simulink model "bu01_2018b"  (R2018b)
settings: Solver=VariableStepAuto  StartTime=0.0  StopTime=10.0  RelTol=1e-3
model workspace (MAT data in the model file):
  Ixx = 0.8
  Iyy = 2.075
  Izz = 1.25
  Mass = 11.5
libraries: aerolibutil x6, sharedtransform x4, simulink x3, sharedutil x3, shared6dof x1
(part 2 of 2)

== system bu01_2018b/bu01_model/推力方程/动力模型/螺旋桨模型1 ==
  u1 : Inport
  Add : Sum  Inputs=4
  Constant : Constant  Value=0
  Constant1 : Constant  Value=0.1591
  Constant2 : Constant  Value=0.1591
  Constant3 : Constant  Value=0.3295
  Constant4 : Constant  Value=0.3295
  Constant5 : Constant  Value=0.7273
  Constant6 : Constant  Value=0.7273
  Constant7 : Constant  Value=1.0
  Gain : Gain  Gain=0.2196
  Gain1 : Gain  Gain=514.4904
  Gain2 : Gain  Gain=2.6589e+03
  Gain3 : Gain  Gain=317.0137
  MATLAB Function : MATLAB Function  TreatAsAtomicUnit=on
  MATLAB Function1 : MATLAB Function  TreatAsAtomicUnit=on
  MATLAB Function2 : MATLAB Function  TreatAsAtomicUnit=on
  MATLAB Function3 : MATLAB Function  TreatAsAtomicUnit=on
  Out1 : Outport
  wires:
  Add/1 -> Out1/1
  u1/1 -> MATLAB Function1/1(u), MATLAB Function/1(u), MATLAB Function2/1(u), MATLAB Function3/1(u)
  Gain3/1 -> Add/4
  Gain2/1 -> Add/3
  Gain1/1 -> Add/2
  Gain/1 -> Add/1
  Constant7/1 -> MATLAB Function3/3(b)
  Constant6/1 -> MATLAB Function3/2(a)
  Constant5/1 -> MATLAB Function2/3(b)
  Constant4/1 -> MATLAB Function2/2(a)
  Constant3/1 -> MATLAB Function1/3(b)
  Constant2/1 -> MATLAB Function1/2(a)
  Constant1/1 -> MATLAB Function/3(b)
  Constant/1 -> MATLAB Function/2(a)
  MATLAB Function3/1(y) -> Gain3/1
  MATLAB Function2/1(y) -> Gain2/1
  MATLAB Function1/1(y) -> Gain1/1
  MATLAB Function/1(y) -> Gain/1

== system bu01_2018b/bu01_model/推力方程/动力模型/螺旋桨模型2 ==
  u1 : Inport
  Add : Sum  Inputs=4
  Constant : Constant  Value=0
  Constant1 : Constant  Value=0.1591
  Constant2 : Constant  Value=0.1591
  Constant3 : Constant  Value=0.3295
  Constant4 : Constant  Value=0.3295
  Constant5 : Constant  Value=0.7273
  Constant6 : Constant  Value=0.7273
  Constant7 : Constant  Value=1.0
  Gain : Gain  Gain=0.2196
  Gain1 : Gain  Gain=514.4904
  Gain2 : Gain  Gain=2.6589e+03
  Gain3 : Gain  Gain=317.0137
  MATLAB Function : MATLAB Function  TreatAsAtomicUnit=on
  MATLAB Function1 : MATLAB Function  TreatAsAtomicUnit=on
  MATLAB Function2 : MATLAB Function  TreatAsAtomicUnit=on
  MATLAB Function3 : MATLAB Function  TreatAsAtomicUnit=on
  Out1 : Outport
  wires:
  MATLAB Function/1(y) -> Gain/1
  MATLAB Function1/1(y) -> Gain1/1
  MATLAB Function2/1(y) -> Gain2/1
  MATLAB Function3/1(y) -> Gain3/1
  Constant/1 -> MATLAB Function/2(a)
  Constant1/1 -> MATLAB Function/3(b)
  Constant2/1 -> MATLAB Function1/2(a)
  Constant3/1 -> MATLAB Function1/3(b)
  Constant4/1 -> MATLAB Function2/2(a)
  Constant5/1 -> MATLAB Function2/3(b)
  Constant6/1 -> MATLAB Function3/2(a)
  Constant7/1 -> MATLAB Function3/3(b)
  Gain/1 -> Add/1
  Gain1/1 -> Add/2
  Gain2/1 -> Add/3
  Gain3/1 -> Add/4
  u1/1 -> MATLAB Function3/1(u), MATLAB Function2/1(u), MATLAB Function/1(u), MATLAB Function1/1(u)
  Add/1 -> Out1/1

== system bu01_2018b/bu01_model/推力方程/动力模型/螺旋桨模型3 ==
  u1 : Inport
  Add : Sum  Inputs=4
  Constant : Constant  Value=0
  Constant1 : Constant  Value=0.1591
  Constant2 : Constant  Value=0.1591
  Constant3 : Constant  Value=0.3295
  Constant4 : Constant  Value=0.3295
  Constant5 : Constant  Value=0.7273
  Constant6 : Constant  Value=0.7273
  Constant7 : Constant  Value=1.0
  Gain : Gain  Gain=0.2196
  Gain1 : Gain  Gain=514.4904
  Gain2 : Gain  Gain=2.6589e+03
  Gain3 : Gain  Gain=317.0137
  MATLAB Function : MATLAB Function  TreatAsAtomicUnit=on
  MATLAB Function1 : MATLAB Function  TreatAsAtomicUnit=on
  MATLAB Function2 : MATLAB Function  TreatAsAtomicUnit=on
  MATLAB Function3 : MATLAB Function  TreatAsAtomicUnit=on
  Out1 : Outport
  wires:
  Add/1 -> Out1/1
  u1/1 -> MATLAB Function1/1(u), MATLAB Function/1(u), MATLAB Function2/1(u), MATLAB Function3/1(u)
  Gain3/1 -> Add/4
  Gain2/1 -> Add/3
  Gain1/1 -> Add/2
  Gain/1 -> Add/1
  Constant7/1 -> MATLAB Function3/3(b)
  Constant6/1 -> MATLAB Function3/2(a)
  Constant5/1 -> MATLAB Function2/3(b)
  Constant4/1 -> MATLAB Function2/2(a)
  Constant3/1 -> MATLAB Function1/3(b)
  Constant2/1 -> MATLAB Function1/2(a)
  Constant1/1 -> MATLAB Function/3(b)
  Constant/1 -> MATLAB Function/2(a)
  MATLAB Function3/1(y) -> Gain3/1
  MATLAB Function2/1(y) -> Gain2/1
  MATLAB Function1/1(y) -> Gain1/1
  MATLAB Function/1(y) -> Gain/1

== system bu01_2018b/bu01_model/推力方程/动力模型/螺旋桨模型4 ==
  u1 : Inport
  Add : Sum  Inputs=4
  Constant : Constant  Value=0
  Constant1 : Constant  Value=0.1591
  Constant2 : Constant  Value=0.1591
  Constant3 : Constant  Value=0.3295
  Constant4 : Constant  Value=0.3295
  Constant5 : Constant  Value=0.7273
  Constant6 : Constant  Value=0.7273
  Constant7 : Constant  Value=1.0
  Gain : Gain  Gain=0.2196
  Gain1 : Gain  Gain=514.4904
  Gain2 : Gain  Gain=2.6589e+03
  Gain3 : Gain  Gain=317.0137
  MATLAB Function : MATLAB Function  TreatAsAtomicUnit=on
  MATLAB Function1 : MATLAB Function  TreatAsAtomicUnit=on
  MATLAB Function2 : MATLAB Function  TreatAsAtomicUnit=on
  MATLAB Function3 : MATLAB Function  TreatAsAtomicUnit=on
  Out1 : Outport
  wires:
  MATLAB Function/1(y) -> Gain/1
  MATLAB Function1/1(y) -> Gain1/1
  MATLAB Function2/1(y) -> Gain2/1
  MATLAB Function3/1(y) -> Gain3/1
  Constant/1 -> MATLAB Function/2(a)
  Constant1/1 -> MATLAB Function/3(b)
  Constant2/1 -> MATLAB Function1/2(a)
  Constant3/1 -> MATLAB Function1/3(b)
  Constant4/1 -> MATLAB Function2/2(a)
  Constant5/1 -> MATLAB Function2/3(b)
  Constant6/1 -> MATLAB Function3/2(a)
  Constant7/1 -> MATLAB Function3/3(b)
  Gain/1 -> Add/1
  Gain1/1 -> Add/2
  Gain2/1 -> Add/3
  Gain3/1 -> Add/4
  u1/1 -> MATLAB Function3/1(u), MATLAB Function2/1(u), MATLAB Function/1(u), MATLAB Function1/1(u)
  Add/1 -> Out1/1

== matlab function bu01_2018b/bu01_model/推力方程/动力模型/螺旋桨模型3/MATLAB Function ==
  data: u input; y output; a input; b input
function y = fst(u,a,b)
    if u>b
        y = 1;
    elseif u<a
        y=0;
    else
        y = (u-a)/(b-a);
    end

== matlab function bu01_2018b/bu01_model/推力方程/动力模型/螺旋桨模型3/MATLAB Function1 ==
  data: u input; y output; a input; b input
function y = fst(u,a,b)
    if u>b
        y = 1;
    elseif u<a
        y=0;
    else
        y = (u-a)/(b-a);
    end

== matlab function bu01_2018b/bu01_model/推力方程/动力模型/螺旋桨模型3/MATLAB Function2 ==
  data: u input; y output; a input; b input
function y = fst(u,a,b)
    if u>b
        y = 1;
    elseif u<a
        y=0;
    else
        y = (u-a)/(b-a);
    end

== matlab function bu01_2018b/bu01_model/推力方程/动力模型/螺旋桨模型3/MATLAB Function3 ==
  data: u input; y output; a input; b input
function y = fst(u,a,b)
    if u>b
        y = 1;
    elseif u<a
        y=0;
    else
        y = (u-a)/(b-a);
    end

== matlab function bu01_2018b/bu01_model/推力方程/动力模型/螺旋桨模型2/MATLAB Function ==
  data: u input; y output; a input; b input
function y = fst(u,a,b)
    if u>b
        y = 1;
    elseif u<a
        y=0;
    else
        y = (u-a)/(b-a);
    end

== matlab function bu01_2018b/bu01_model/推力方程/动力模型/螺旋桨模型2/MATLAB Function1 ==
  data: u input; y output; a input; b input
function y = fst(u,a,b)
    if u>b
        y = 1;
    elseif u<a
        y=0;
    else
        y = (u-a)/(b-a);
    end

== matlab function bu01_2018b/bu01_model/推力方程/动力模型/涵道模型模型2/MATLAB Function ==
  data: u input; y output; a input; b input
function y = fst(u,a,b)
    if u>b
        y = 1;
    elseif u<a
        y=0;
    else
        y = (u-a)/(b-a);
    end

== matlab function bu01_2018b/bu01_model/推力方程/动力模型/涵道模型模型2/MATLAB Function1 ==
  data: u input; y output; a input; b input
function y = fst(u,a,b)
    if u>b
        y = 1;
    elseif u<a
        y=0;
    else
        y = (u-a)/(b-a);
    end

== matlab function bu01_2018b/bu01_model/推力方程/动力模型/螺旋桨模型2/MATLAB Function2 ==
  data: u input; y output; a input; b input
function y = fst(u,a,b)
    if u>b
        y = 1;
    elseif u<a
        y=0;
    else
        y = (u-a)/(b-a);
    end

== matlab function bu01_2018b/bu01_model/推力方程/动力模型/螺旋桨模型2/MATLAB Function3 ==
  data: u input; y output; a input; b input
function y = fst(u,a,b)
    if u>b
        y = 1;
    elseif u<a
        y=0;
    else
        y = (u-a)/(b-a);
    end

== matlab function bu01_2018b/bu01_model/推力方程/动力模型/螺旋桨模型4/MATLAB Function ==
  data: u input; y output; a input; b input
function y = fst(u,a,b)
    if u>b
        y = 1;
    elseif u<a
        y=0;
    else
        y = (u-a)/(b-a);
    end

== matlab function bu01_2018b/bu01_model/推力方程/动力模型/螺旋桨模型4/MATLAB Function1 ==
  data: u input; y output; a input; b input
function y = fst(u,a,b)
    if u>b
        y = 1;
    elseif u<a
        y=0;
    else
        y = (u-a)/(b-a);
    end

== matlab function bu01_2018b/bu01_model/推力方程/动力模型/螺旋桨模型4/MATLAB Function2 ==
  data: u input; y output; a input; b input
function y = fst(u,a,b)
    if u>b
        y = 1;
    elseif u<a
        y=0;
    else
        y = (u-a)/(b-a);
    end

== matlab function bu01_2018b/bu01_model/推力方程/动力模型/螺旋桨模型4/MATLAB Function3 ==
  data: u input; y output; a input; b input
function y = fst(u,a,b)
    if u>b
        y = 1;
    elseif u<a
        y=0;
    else
        y = (u-a)/(b-a);
    end

== matlab function bu01_2018b/bu01_model/推力方程/动力模型/涵道模型模型1/MATLAB Function ==
  data: u input; y output; a input; b input
function y = fst(u,a,b)
    if u>b
        y = 1;
    elseif u<a
        y=0;
    else
        y = (u-a)/(b-a);
    end

== matlab function bu01_2018b/bu01_model/推力方程/动力模型/涵道模型模型1/MATLAB Function1 ==
  data: u input; y output; a input; b input
function y = fst(u,a,b)
    if u>b
        y = 1;
    elseif u<a
        y=0;
    else
        y = (u-a)/(b-a);
    end

== matlab function bu01_2018b/bu01_model/推力方程/动力模型/涵道模型模型3/MATLAB Function ==
  data: u input; y output; a input; b input
function y = fst(u,a,b)
    if u>b
        y = 1;
    elseif u<a
        y=0;
    else
        y = (u-a)/(b-a);
    end

== matlab function bu01_2018b/bu01_model/推力方程/动力模型/涵道模型模型3/MATLAB Function1 ==
  data: u input; y output; a input; b input
function y = fst(u,a,b)
    if u>b
        y = 1;
    elseif u<a
        y=0;
    else
        y = (u-a)/(b-a);
    end

== matlab function bu01_2018b/bu01_model/推力方程/动力模型/螺旋桨模型1/MATLAB Function ==
  data: u input; y output; a input; b input
function y = fst(u,a,b)
    if u>b
        y = 1;
    elseif u<a
        y=0;
    else
        y = (u-a)/(b-a);
    end

== matlab function bu01_2018b/bu01_model/推力方程/动力模型/螺旋桨模型1/MATLAB Function1 ==
  data: u input; y output; a input; b input
function y = fst(u,a,b)
    if u>b
        y = 1;
    elseif u<a
        y=0;
    else
        y = (u-a)/(b-a);
    end

== matlab function bu01_2018b/bu01_model/推力方程/动力模型/螺旋桨模型1/MATLAB Function2 ==
  data: u input; y output; a input; b input
function y = fst(u,a,b)
    if u>b
        y = 1;
    elseif u<a
        y=0;
    else
        y = (u-a)/(b-a);
    end

== matlab function bu01_2018b/bu01_model/推力方程/动力模型/螺旋桨模型1/MATLAB Function3 ==
  data: u input; y output; a input; b input
function y = fst(u,a,b)
    if u>b
        y = 1;
    elseif u<a
        y=0;
    else
        y = (u-a)/(b-a);
    end

== matlab function bu01_2018b/bu01_model/推力方程/动力模型/涵道模型模型4/MATLAB Function ==
  data: u input; y output; a input; b input
function y = fst(u,a,b)
    if u>b
        y = 1;
    elseif u<a
        y=0;
    else
        y = (u-a)/(b-a);
    end

== matlab function bu01_2018b/bu01_model/推力方程/动力模型/涵道模型模型4/MATLAB Function1 ==
  data: u input; y output; a input; b input
function y = fst(u,a,b)
    if u>b
        y = 1;
    elseif u<a
        y=0;
    else
        y = (u-a)/(b-a);
    end

== matlab function bu01_2018b/bu01_model/力矩方程/推力模型/涵道模型模型1/MATLAB Function ==
  data: u input; y output; a input; b input
function y = fst(u,a,b)
    if u>b
        y = 1;
    elseif u<a
        y=0;
    else
        y = (u-a)/(b-a);
    end

== matlab function bu01_2018b/bu01_model/力矩方程/推力模型/涵道模型模型1/MATLAB Function1 ==
  data: u input; y output; a input; b input
function y = fst(u,a,b)
    if u>b
        y = 1;
    elseif u<a
        y=0;
    else
        y = (u-a)/(b-a);
    end

== matlab function bu01_2018b/bu01_model/力矩方程/推力模型/涵道模型模型2/MATLAB Function ==
  data: u input; y output; a input; b input
function y = fst(u,a,b)
    if u>b
        y = 1;
    elseif u<a
        y=0;
    else
        y = (u-a)/(b-a);
    end

== matlab function bu01_2018b/bu01_model/力矩方程/推力模型/涵道模型模型2/MATLAB Function1 ==
  data: u input; y output; a input; b input
function y = fst(u,a,b)
    if u>b
        y = 1;
    elseif u<a
        y=0;
    else
        y = (u-a)/(b-a);
    end

== matlab function bu01_2018b/bu01_model/力矩方程/推力模型/涵道模型模型3/MATLAB Function ==
  data: u input; y output; a input; b input
function y = fst(u,a,b)
    if u>b
        y = 1;
    elseif u<a
        y=0;
    else
        y = (u-a)/(b-a);
    end

== matlab function bu01_2018b/bu01_model/力矩方程/推力模型/涵道模型模型3/MATLAB Function1 ==
  data: u input; y output; a input; b input
function y = fst(u,a,b)
    if u>b
        y = 1;
    elseif u<a
        y=0;
    else
        y = (u-a)/(b-a);
    end

== matlab function bu01_2018b/bu01_model/力矩方程/推力模型/涵道模型模型4/MATLAB Function ==
  data: u input; y output; a input; b input
function y = fst(u,a,b)
    if u>b
        y = 1;
    elseif u<a
        y=0;
    else
        y = (u-a)/(b-a);
    end

== matlab function bu01_2018b/bu01_model/力矩方程/推力模型/涵道模型模型4/MATLAB Function1 ==
  data: u input; y output; a input; b input
function y = fst(u,a,b)
    if u>b
        y = 1;
    elseif u<a
        y=0;
    else
        y = (u-a)/(b-a);
    end

== matlab function bu01_2018b/bu01_model/力矩方程/推力模型/螺旋桨模型1/MATLAB Function ==
  data: u input; y output; a input; b input
function y = fst(u,a,b)
    if u>b
        y = 1;
    elseif u<a
        y=0;
    else
        y = (u-a)/(b-a);
    end

== matlab function bu01_2018b/bu01_model/力矩方程/推力模型/螺旋桨模型1/MATLAB Function1 ==
  data: u input; y output; a input; b input
function y = fst(u,a,b)
    if u>b
        y = 1;
    elseif u<a
        y=0;
    else
        y = (u-a)/(b-a);
    end

== matlab function bu01_2018b/bu01_model/力矩方程/推力模型/螺旋桨模型1/MATLAB Function2 ==
  data: u input; y output; a input; b input
function y = fst(u,a,b)
    if u>b
        y = 1;
    elseif u<a
        y=0;
    else
        y = (u-a)/(b-a);
    end

== matlab function bu01_2018b/bu01_model/力矩方程/推力模型/螺旋桨模型1/MATLAB Function3 ==
  data: u input; y output; a input; b input
function y = fst(u,a,b)
    if u>b
        y = 1;
    elseif u<a
        y=0;
    else
        y = (u-a)/(b-a);
    end

== matlab function bu01_2018b/bu01_model/力矩方程/推力模型/螺旋桨模型2/MATLAB Function ==
  data: u input; y output; a input; b input
function y = fst(u,a,b)
    if u>b
        y = 1;
    elseif u<a
        y=0;
    else
        y = (u-a)/(b-a);
    end

== matlab function bu01_2018b/bu01_model/力矩方程/推力模型/螺旋桨模型2/MATLAB Function1 ==
  data: u input; y output; a input; b input
function y = fst(u,a,b)
    if u>b
        y = 1;
    elseif u<a
        y=0;
    else
        y = (u-a)/(b-a);
    end

== matlab function bu01_2018b/bu01_model/力矩方程/推力模型/螺旋桨模型2/MATLAB Function2 ==
  data: u input; y output; a input; b input
function y = fst(u,a,b)
    if u>b
        y = 1;
    elseif u<a
        y=0;
    else
        y = (u-a)/(b-a);
    end

== matlab function bu01_2018b/bu01_model/力矩方程/推力模型/螺旋桨模型2/MATLAB Function3 ==
  data: u input; y output; a input; b input
function y = fst(u,a,b)
    if u>b
        y = 1;
    elseif u<a
        y=0;
    else
        y = (u-a)/(b-a);
    end

== matlab function bu01_2018b/bu01_model/力矩方程/推力模型/螺旋桨模型3/MATLAB Function ==
  data: u input; y output; a input; b input
function y = fst(u,a,b)
    if u>b
        y = 1;
    elseif u<a
        y=0;
    else
        y = (u-a)/(b-a);
    end

== matlab function bu01_2018b/bu01_model/力矩方程/推力模型/螺旋桨模型3/MATLAB Function1 ==
  data: u input; y output; a input; b input
function y = fst(u,a,b)
    if u>b
        y = 1;
    elseif u<a
        y=0;
    else
        y = (u-a)/(b-a);
    end

== matlab function bu01_2018b/bu01_model/力矩方程/推力模型/螺旋桨模型3/MATLAB Function2 ==
  data: u input; y output; a input; b input
function y = fst(u,a,b)
    if u>b
        y = 1;
    elseif u<a
        y=0;
    else
        y = (u-a)/(b-a);
    end

== matlab function bu01_2018b/bu01_model/力矩方程/推力模型/螺旋桨模型3/MATLAB Function3 ==
  data: u input; y output; a input; b input
function y = fst(u,a,b)
    if u>b
        y = 1;
    elseif u<a
        y=0;
    else
        y = (u-a)/(b-a);
    end

== matlab function bu01_2018b/bu01_model/力矩方程/推力模型/螺旋桨模型4/MATLAB Function ==
  data: u input; y output; a input; b input
function y = fst(u,a,b)
    if u>b
        y = 1;
    elseif u<a
        y=0;
    else
        y = (u-a)/(b-a);
    end

== matlab function bu01_2018b/bu01_model/力矩方程/推力模型/螺旋桨模型4/MATLAB Function1 ==
  data: u input; y output; a input; b input
function y = fst(u,a,b)
    if u>b
        y = 1;
    elseif u<a
        y=0;
    else
        y = (u-a)/(b-a);
    end

== matlab function bu01_2018b/bu01_model/力矩方程/推力模型/螺旋桨模型4/MATLAB Function2 ==
  data: u input; y output; a input; b input
function y = fst(u,a,b)
    if u>b
        y = 1;
    elseif u<a
        y=0;
    else
        y = (u-a)/(b-a);
    end

== matlab function bu01_2018b/bu01_model/力矩方程/推力模型/螺旋桨模型4/MATLAB Function3 ==
  data: u input; y output; a input; b input
function y = fst(u,a,b)
    if u>b
        y = 1;
    elseif u<a
        y=0;
    else
        y = (u-a)/(b-a);
    end

== matlab function bu01_2018b/bu01_model/力矩方程/扭力模型/螺旋桨模型1/MATLAB Function ==
  data: u input; y output; a input; b input
function y = fst(u,a,b)
    if u>b
        y = 1;
    elseif u<a
        y=0;
    else
        y = (u-a)/(b-a);
    end

== matlab function bu01_2018b/bu01_model/力矩方程/扭力模型/螺旋桨模型1/MATLAB Function1 ==
  data: u input; y output; a input; b input
function y = fst(u,a,b)
    if u>b
        y = 1;
    elseif u<a
        y=0;
    else
        y = (u-a)/(b-a);
    end

== matlab function bu01_2018b/bu01_model/力矩方程/扭力模型/螺旋桨模型1/MATLAB Function2 ==
  data: u input; y output; a input; b input
function y = fst(u,a,b)
    if u>b
        y = 1;
    elseif u<a
        y=0;
    else
        y = (u-a)/(b-a);
    end

== matlab function bu01_2018b/bu01_model/力矩方程/扭力模型/螺旋桨模型1/MATLAB Function3 ==
  data: u input; y output; a input; b input
function y = fst(u,a,b)
    if u>b
        y = 1;
    elseif u<a
        y=0;
    else
        y = (u-a)/(b-a);
    end

== matlab function bu01_2018b/bu01_model/力矩方程/扭力模型/涵道模型模型1/MATLAB Function ==
  data: u input; y output; a input; b input
function y = fst(u,a,b)
    if u>b
        y = 1;
    elseif u<a
        y=0;
    else
        y = (u-a)/(b-a);
    end

== matlab function bu01_2018b/bu01_model/力矩方程/扭力模型/涵道模型模型1/MATLAB Function1 ==
  data: u input; y output; a input; b input
function y = fst(u,a,b)
    if u>b
        y = 1;
    elseif u<a
        y=0;
    else
        y = (u-a)/(b-a);
    end

== matlab function bu01_2018b/bu01_model/力矩方程/扭力模型/螺旋桨模型2/MATLAB Function ==
  data: u input; y output; a input; b input
function y = fst(u,a,b)
    if u>b
        y = 1;
    elseif u<a
        y=0;
    else
        y = (u-a)/(b-a);
    end

== matlab function bu01_2018b/bu01_model/力矩方程/扭力模型/螺旋桨模型2/MATLAB Function1 ==
  data: u input; y output; a input; b input
function y = fst(u,a,b)
    if u>b
        y = 1;
    elseif u<a
        y=0;
    else
        y = (u-a)/(b-a);
    end

== matlab function bu01_2018b/bu01_model/力矩方程/扭力模型/螺旋桨模型2/MATLAB Function2 ==
  data: u input; y output; a input; b input
function y = fst(u,a,b)
    if u>b
        y = 1;
    elseif u<a
        y=0;
    else
        y = (u-a)/(b-a);
    end

== matlab function bu01_2018b/bu01_model/力矩方程/扭力模型/螺旋桨模型2/MATLAB Function3 ==
  data: u input; y output; a input; b input
function y = fst(u,a,b)
    if u>b
        y = 1;
    elseif u<a
        y=0;
    else
        y = (u-a)/(b-a);
    end

== matlab function bu01_2018b/bu01_model/力矩方程/扭力模型/涵道模型模型2/MATLAB Function ==
  data: u input; y output; a input; b input
function y = fst(u,a,b)
    if u>b
        y = 1;
    elseif u<a
        y=0;
    else
        y = (u-a)/(b-a);
    end

== matlab function bu01_2018b/bu01_model/力矩方程/扭力模型/涵道模型模型2/MATLAB Function1 ==
  data: u input; y output; a input; b input
function y = fst(u,a,b)
    if u>b
        y = 1;
    elseif u<a
        y=0;
    else
        y = (u-a)/(b-a);
    end

== matlab function bu01_2018b/bu01_model/力矩方程/扭力模型/涵道模型模型3/MATLAB Function ==
  data: u input; y output; a input; b input
function y = fst(u,a,b)
    if u>b
        y = 1;
    elseif u<a
        y=0;
    else
        y = (u-a)/(b-a);
    end

== matlab function bu01_2018b/bu01_model/力矩方程/扭力模型/涵道模型模型3/MATLAB Function1 ==
  data: u input; y output; a input; b input
function y = fst(u,a,b)
    if u>b
        y = 1;
    elseif u<a
        y=0;
    else
        y = (u-a)/(b-a);
    end

== matlab function bu01_2018b/bu01_model/力矩方程/扭力模型/涵道模型模型4/MATLAB Function ==
  data: u input; y output; a input; b input
function y = fst(u,a,b)
    if u>b
        y = 1;
    elseif u<a
        y=0;
    else
        y = (u-a)/(b-a);
    end

== matlab function bu01_2018b/bu01_model/力矩方程/扭力模型/涵道模型模型4/MATLAB Function1 ==
  data: u input; y output; a input; b input
function y = fst(u,a,b)
    if u>b
        y = 1;
    elseif u<a
        y=0;
    else
        y = (u-a)/(b-a);
    end

== matlab function bu01_2018b/bu01_model/力矩方程/扭力模型/螺旋桨模型3/MATLAB Function ==
  data: u input; y output; a input; b input
function y = fst(u,a,b)
    if u>b
        y = 1;
    elseif u<a
        y=0;
    else
        y = (u-a)/(b-a);
    end

== matlab function bu01_2018b/bu01_model/力矩方程/扭力模型/螺旋桨模型3/MATLAB Function1 ==
  data: u input; y output; a input; b input
function y = fst(u,a,b)
    if u>b
        y = 1;
    elseif u<a
        y=0;
    else
        y = (u-a)/(b-a);
    end

== matlab function bu01_2018b/bu01_model/力矩方程/扭力模型/螺旋桨模型3/MATLAB Function2 ==
  data: u input; y output; a input; b input
function y = fst(u,a,b)
    if u>b
        y = 1;
    elseif u<a
        y=0;
    else
        y = (u-a)/(b-a);
    end

== matlab function bu01_2018b/bu01_model/力矩方程/扭力模型/螺旋桨模型3/MATLAB Function3 ==
  data: u input; y output; a input; b input
function y = fst(u,a,b)
    if u>b
        y = 1;
    elseif u<a
        y=0;
    else
        y = (u-a)/(b-a);
    end

== matlab function bu01_2018b/bu01_model/力矩方程/扭力模型/螺旋桨模型4/MATLAB Function ==
  data: u input; y output; a input; b input
function y = fst(u,a,b)
    if u>b
        y = 1;
    elseif u<a
        y=0;
    else
        y = (u-a)/(b-a);
    end

== matlab function bu01_2018b/bu01_model/力矩方程/扭力模型/螺旋桨模型4/MATLAB Function1 ==
  data: u input; y output; a input; b input
function y = fst(u,a,b)
    if u>b
        y = 1;
    elseif u<a
        y=0;
    else
        y = (u-a)/(b-a);
    end

== matlab function bu01_2018b/bu01_model/力矩方程/扭力模型/螺旋桨模型4/MATLAB Function2 ==
  data: u input; y output; a input; b input
function y = fst(u,a,b)
    if u>b
        y = 1;
    elseif u<a
        y=0;
    else
        y = (u-a)/(b-a);
    end

== matlab function bu01_2018b/bu01_model/力矩方程/扭力模型/螺旋桨模型4/MATLAB Function3 ==
  data: u input; y output; a input; b input
function y = fst(u,a,b)
    if u>b
        y = 1;
    elseif u<a
        y=0;
    else
        y = (u-a)/(b-a);
    end

== matlab function bu01_2018b/控制器/求取航向衰减后的期望四元数/MATLAB Function ==
  data: src input; q output; dst input
function q = vec2quat(src, dst)
    quat = [1 0 0 0];
    cr = cross(src, dst);
    dt = dot(src, dst);
    % 处理向量夹角为180度的情况
    if norm(cr) < eps && dt < 0
       cr = abs(src);
       if cr(1) < cr(2)
          if cr(1) < cr(3)
              cr = [1 0 0];
          else
              cr = [0 0 1];
          end
       else
           if cr(2) < cr(3)
               cr = [0 1 0];
           else
               cr = [0 0 1];
           end
       end
       quat(1) = 0;
       cr = cross(src, cr);
    else
        quat(1) = dt + norm(src)*norm(dst);
    end
    quat(2) = cr(1);
    quat(3) = cr(2);
    quat(4) = cr(3);
    q = quat;
